simulink model "Electric_Machines_Design"  (R2021a)
settings: Solver=ode4  StartTime=0.0  StopTime=10.0  FixedStep=1e-6  RelTol=1e-3
libraries: spsSeriesRLCBranchLib x14, spsVoltageMeasurementLib x4, spsRMSLib x3, spsACVoltageSourceLib x1, spsAsynchronousMachineSIUnitsLib x1, spsPWMGenerator2LevelLib x1, spsTwoLevelConverterLib x1, spsUniversalBridgeLib x1, spsVariableRatioTransformerLib x1, spspowerguiLib x1
settings Model: Creator=SULEYMAN  LastModifiedBy=erena
settings DebuggingCC: UnconnectedInputMsg=none  UnconnectedOutputMsg=none  UnconnectedLineMsg=none
settings ModelReferenceCC: EnableRefExpFcnMdlSchedulingChecks=off
settings RTWCC: Description=Generic Real-Time Target  GPUComputeCapability=5.0  DLArmComputeVersion=20.02.1

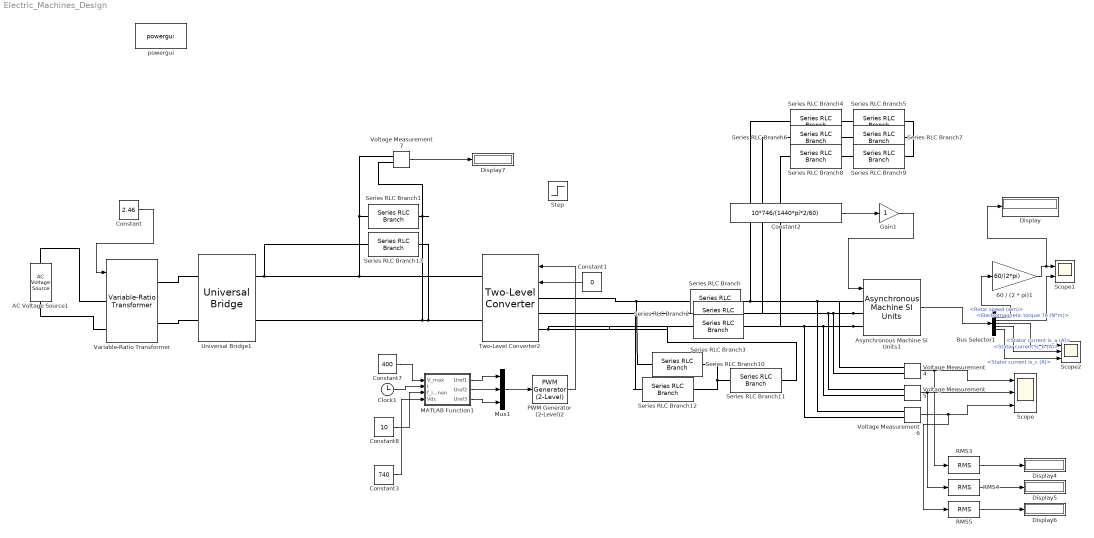
== system Electric_Machines_Design ==
  60 / (2 * pi)1 : Gain  Gain=60/(2*pi)
  AC Voltage Source1 : spsACVoltageSourceLib/AC Voltage Source  Amplitude=312  Phase=0  Frequency=50  SampleTime=0  Measurements=None  BusType=swing  Pref=10e3  Qref=0  Qmin=-inf  Qmax=+inf
  Asynchronous Machine SI Units1 : spsAsynchronousMachineSIUnitsLib/Asynchronous Machine SI Units  RotorType=Squirrel-cage  PresetModel="16:  10 HP (7.5KW)  400 V 50Hz 1440 RPM"  MechanicalLoad=Torque Tm  ShowDetailedParameters=on  ReferenceFrame=Rotor  Units=SI  MeasurementBus=off  NominalParameters=[7500 400 50]  VoltageRatio=1  Stator=[0.7384 0.003045]  Rotor=[0.7402 0.003045]  Cage1=[0.4155 0.002066]  Cage2=[0.4168 0.0003495]  Lm=0.1241  Mechanical=[0.0343 0.000503 2]  PolePairs=2  InitialConditions=[1 0 0 0 0 0 0 0]  SimulateSaturation=off  Saturation=[14.03593122, 27.81365428, 53.79336849, 72.68890987, 97.98006896, 148.6815601, 215.7428561, 302.9841135, 428.7778367 ; 230, 322, 414, 460, 506, 552, 598, 644, 690]  LoadFlowParameters=1492000  TsPowergui=0  TsBlock=-1  IterativeModel=Trapezoidal non iterative  IterativeDiscreteModel=Trapezoidal non iterative  Pmec=1.492e+006
  Bus Selector1 : BusSelector  OutputSignals=Mechanical.Rotor speed (wm),Mechanical.Electromagnetic torque Te (N*m),Stator measurements.Stator current is_a (A),Stator measurements.Stator current is_b (A),Stator measurements.Stator current is_c (A)
  Clock1 : Clock
  Constant : Constant  Value=2.46
  Constant1 : Constant  Value=0
  Constant2 : Constant  Value=10*746/(1440*pi*2/60)
  Constant3 : Constant  Value=740
  Constant7 : Constant  Value=400
  Constant8 : Constant  Value=10
  Display{,4..7} (5 alike) : Display
      Display6 settings: Decimation=50
  Gain1 : Gain
  MATLAB Function1 : MATLAB Function  TreatAsAtomicUnit=on
  Mux1 : Mux  Inputs=3
  PWM Generator (2-Level)2 : spsPWMGenerator2LevelLib/PWM Generator (2-Level)  ModulatorType=Three-phase bridge (6 pulses)  ModulatorMode=Unsynchronized  Fc=200*60  Pc=90  nF=27  MinMax="[ -1  1 ]"  SamplingTechnique=Natural  ModulatingSignals=off  m=0.8  Freq=60  Phase=0  Ts=1e-6  ShowCarrierOutport=off
  RMS3 : spsRMSLib/RMS  TrueRMS=off  Freq=10  RMSInit=0  Ts=0
  RMS4 : spsRMSLib/RMS  TrueRMS=off  Freq=10  RMSInit=0  Ts=0
  RMS5 : spsRMSLib/RMS  TrueRMS=off  Freq=10  RMSInit=0  Ts=0
  Scope : Scope  NumInputPorts=3
  Scope1 : Scope  NumInputPorts=2
  Scope2 : Scope  NumInputPorts=3
  Series RLC Branch : spsSeriesRLCBranchLib/Series RLC Branch  LConnTagsString=__new0  RConnTagsString=__new0  BranchType=L  Resistance=1  Inductance=3.5e-3  SetiL0=off  InitialCurrent=0  Capacitance=1e-6  Setx0=off  InitialVoltage=0  Measurements=None
  Series RLC Branch1 : spsSeriesRLCBranchLib/Series RLC Branch  LConnTagsString=__new0  RConnTagsString=__new0  BranchType=C  Resistance=1  Inductance=1e-3  SetiL0=off  InitialCurrent=0  Capacitance=4700e-6  Setx0=off  InitialVoltage=0  Measurements=None
  Series RLC Branch10 : spsSeriesRLCBranchLib/Series RLC Branch  LConnTagsString=__new0  RConnTagsString=__new0  BranchType=R  Resistance=1e5  Inductance=1e-3  SetiL0=off  InitialCurrent=0  Capacitance=1e-6  Setx0=off  InitialVoltage=0  Measurements=None
  Series RLC Branch11 : spsSeriesRLCBranchLib/Series RLC Branch  LConnTagsString=__new0  RConnTagsString=__new0  BranchType=R  Resistance=1e5  Inductance=1e-3  SetiL0=off  InitialCurrent=0  Capacitance=1e-6  Setx0=off  InitialVoltage=0  Measurements=None
  Series RLC Branch12 : spsSeriesRLCBranchLib/Series RLC Branch  LConnTagsString=__new0  RConnTagsString=__new0  BranchType=R  Resistance=1e5  Inductance=1e-3  SetiL0=off  InitialCurrent=0  Capacitance=1e-6  Setx0=off  InitialVoltage=0  Measurements=None
  Series RLC Branch13 : spsSeriesRLCBranchLib/Series RLC Branch  LConnTagsString=__new0  RConnTagsString=__new0  BranchType=C  Resistance=1  Inductance=1e-3  SetiL0=off  InitialCurrent=0  Capacitance=4700e-6  Setx0=off  InitialVoltage=0  Measurements=None
  Series RLC Branch2 : spsSeriesRLCBranchLib/Series RLC Branch  LConnTagsString=__new0  RConnTagsString=__new0  BranchType=L  Resistance=1  Inductance=3.5e-3  SetiL0=off  InitialCurrent=0  Capacitance=1e-6  Setx0=off  InitialVoltage=0  Measurements=None
  Series RLC Branch3 : spsSeriesRLCBranchLib/Series RLC Branch  LConnTagsString=__new0  RConnTagsString=__new0  BranchType=L  Resistance=1  Inductance=3.5e-3  SetiL0=off  InitialCurrent=0  Capacitance=1e-6  Setx0=off  InitialVoltage=0  Measurements=None
  Series RLC Branch4 : spsSeriesRLCBranchLib/Series RLC Branch  LConnTagsString=__new0  RConnTagsString=__new0  BranchType=C  Resistance=1  Inductance=1e-3  SetiL0=off  InitialCurrent=0  Capacitance=6.6e-6  Setx0=off  InitialVoltage=0  Measurements=None
  Series RLC Branch5 : spsSeriesRLCBranchLib/Series RLC Branch  LConnTagsString=__new0  RConnTagsString=__new0  BranchType=R  Resistance=5  Inductance=1e-3  SetiL0=off  InitialCurrent=0  Capacitance=1e-6  Setx0=off  InitialVoltage=0  Measurements=None
  Series RLC Branch6 : spsSeriesRLCBranchLib/Series RLC Branch  LConnTagsString=__new0  RConnTagsString=__new0  BranchType=C  Resistance=1  Inductance=1e-3  SetiL0=off  InitialCurrent=0  Capacitance=6.6e-6  Setx0=off  InitialVoltage=0  Measurements=None
  Series RLC Branch7 : spsSeriesRLCBranchLib/Series RLC Branch  LConnTagsString=__new0  RConnTagsString=__new0  BranchType=R  Resistance=5  Inductance=1e-3  SetiL0=off  InitialCurrent=0  Capacitance=1e-6  Setx0=off  InitialVoltage=0  Measurements=None
  Series RLC Branch8 : spsSeriesRLCBranchLib/Series RLC Branch  LConnTagsString=__new0  RConnTagsString=__new0  BranchType=C  Resistance=1  Inductance=1e-3  SetiL0=off  InitialCurrent=0  Capacitance=6.6e-6  Setx0=off  InitialVoltage=0  Measurements=None
  Series RLC Branch9 : spsSeriesRLCBranchLib/Series RLC Branch  LConnTagsString=__new0  RConnTagsString=__new0  BranchType=R  Resistance=5  Inductance=1e-3  SetiL0=off  InitialCurrent=0  Capacitance=1e-6  Setx0=off  InitialVoltage=0  Measurements=None
  Step : Step  Time=2.5  After=10*746/(1440*pi*2/60)  SampleTime=0
  Two-Level Converter2 : spsTwoLevelConverterLib/Two-Level Converter  ModelType=Switching devices  Ron=1e-3  Rs=1e6  Cs=inf  Vforward=[0,0]  Ron_Diode=1e-3  Rs_Diode=1e6  Cs_Diode=inf  Vf_Diode=1e-3  Rs_CurrentSource=inf
      settings: SourceProductBaseCode=PS
  Universal Bridge1 : spsUniversalBridgeLib/Universal Bridge  Arms=2  SnubberResistance=1e5  SnubberCapacitance=inf  Device=Diodes  Ron=1e-3  Lon=0  ForwardVoltages="[  0  0  ]"  ForwardVoltage=0  GTOparameters=[ 10e-6 , 20e-6 ]  IGBTparameters=[ 1e-6 , 2e-6 ]  Measurements=None  Measurements_2=None  converterType=Rectifier
  Variable-Ratio Transformer : spsVariableRatioTransformerLib/Variable-Ratio Transformer
      settings: SourceProductBaseCode=PS
  Voltage Measurement{4..7} (4 alike) : spsVoltageMeasurementLib/Voltage Measurement  PhasorSimulation=off  OutputType=Complex  PSBequivalent=0
  powergui : spspowerguiLib/powergui  Priority=1  SimulationMode=Discrete  SampleTime=1e-6  frequency=50  Iterations=50  frequencyindice=50  Pbase=100e6  ErrMax=1e-4  UnitsV=kV  UnitsW=MW  buscounter=0  FunctionMessages=off  echomessages=off  EnableUseOfTLC=off  CurrentSourceSwitches=off  DisableSnubberDevices=off  DisableRonSwitches=off  DisableVfSwitches=off  DisplayEquations=off  AutomaticDiscreteSolvers=off  SolverType=Tustin/Backward Euler (TBE)  Interpol=off  ExternalGateDelay=off  methode=off  Ts=100  x0status=blocks  SPID=on  SwTol=0  HookPort=off  NonlinearTolerance=1e-4  nMaxIteration=100  ContinueOnMaxIteration=off  RestoreLinks=warning  ResistiveCurrentMeasurement=off  Frange=[0:2:500]  Ylog=off  Xlog=on  ShowGrid=off  save=off  variable=ZData  structure=0  ZoomFFT=off  StartTime=0.0  cycles=1  DisplayStyle=1  fundamental=60  FreqAxis=off  MaxFrequency=1000  frequencyindicesteady=1  RmsSteady=1  display=off
  wires:
  Asynchronous Machine SI Units1/1 -> Bus Selector1/1
  MATLAB Function1/1(Uref1) -> Mux1/1
  Voltage Measurement7/1 -> Display7/1
  Bus Selector1/4 -> Scope2/2  "<Stator current is_b (A)>"
  60 / (2 * pi)1/1 -> Display/1, Scope1/1
  Bus Selector1/3 -> Scope2/1  "<Stator current is_a (A)>"
  Bus Selector1/2 -> Scope1/2  "<Electromagnetic torque Te (N*m)>"
  Constant1/1 -> Two-Level Converter2/2
  PWM Generator (2-Level)2/1 -> Two-Level Converter2/1
  MATLAB Function1/3(Uref3) -> Mux1/3
  Bus Selector1/5 -> Scope2/3  "<Stator current is_c (A)>"
  Clock1/1 -> MATLAB Function1/2(t)
  Bus Selector1/1 -> 60 / (2 * pi)1/1  "<Rotor speed (wm)>"
  Constant7/1 -> MATLAB Function1/1(V_max)
  Mux1/1 -> PWM Generator (2-Level)2/1
  Gain1/1 -> Asynchronous Machine SI Units1/1
  MATLAB Function1/2(Uref2) -> Mux1/2
  Constant/1 -> Variable-Ratio Transformer/1
  RMS3/1 -> Display4/1
  RMS4/1 -> Display5/1
  RMS5/1 -> Display6/1
  Voltage Measurement4/1 -> Scope/1, RMS3/1
  Voltage Measurement5/1 -> Scope/2, RMS4/1
  Voltage Measurement6/1 -> RMS5/1, Scope/3
  Constant8/1 -> MATLAB Function1/3(f_istenen)
  Constant3/1 -> MATLAB Function1/4(Vdc)
  Constant2/1 -> Gain1/1
  connections:
  Asynchronous Machine SI Units1/LConn3 -- Voltage Measurement6/LConn2 -- Series RLC Branch8/LConn1 -- Series RLC Branch3/RConn1 -- Voltage Measurement5/LConn2
  Asynchronous Machine SI Units1/LConn1 -- Voltage Measurement4/LConn1 -- Voltage Measurement6/LConn1 -- Series RLC Branch4/LConn1 -- Series RLC Branch/RConn1
  Series RLC Branch1/RConn1 -- Voltage Measurement7/LConn2 -- Series RLC Branch13/RConn1 -- Two-Level Converter2/RConn2 -- Universal Bridge1/RConn2
  Asynchronous Machine SI Units1/LConn2 -- Voltage Measurement4/LConn2 -- Series RLC Branch6/LConn1 -- Series RLC Branch2/RConn1 -- Voltage Measurement5/LConn1
  AC Voltage Source1/RConn1 -- Variable-Ratio Transformer/LConn1
  AC Voltage Source1/LConn1 -- Variable-Ratio Transformer/LConn2
  Universal Bridge1/LConn1 -- Variable-Ratio Transformer/RConn1
  Variable-Ratio Transformer/RConn2 -- Universal Bridge1/LConn2
  Series RLC Branch/LConn1 -- Series RLC Branch10/LConn1 -- Two-Level Converter2/LConn1
  Two-Level Converter2/LConn2 -- Series RLC Branch12/LConn1 -- Series RLC Branch2/LConn1
  Two-Level Converter2/LConn3 -- Series RLC Branch11/LConn1 -- Series RLC Branch3/LConn1
  Series RLC Branch4/RConn1 -- Series RLC Branch5/LConn1
  Series RLC Branch6/RConn1 -- Series RLC Branch7/LConn1
  Series RLC Branch8/RConn1 -- Series RLC Branch9/LConn1
  Series RLC Branch5/RConn1 -- Series RLC Branch9/RConn1 -- Series RLC Branch7/RConn1
  Series RLC Branch10/RConn1 -- Series RLC Branch11/RConn1 -- Series RLC Branch12/RConn1
  Series RLC Branch1/LConn1 -- Voltage Measurement7/LConn1 -- Series RLC Branch13/LConn1 -- Universal Bridge1/RConn1 -- Two-Level Converter2/RConn1

== matlab function Electric_Machines_Design/MATLAB Function1 ==
  settings: updateMethod=DISCRETE
  data: V_max input; t input; f_istenen input; Uref1 output; Uref2 output; Uref3 output; Vdc input
function [Uref1, Uref2, Uref3] = fcn(V_max, t, f_istenen, Vdc)

    % Hertz başına 8 Volt artış kuralı
    volt_per_hz = 8;
    V_ref = volt_per_hz * f_istenen; 

    % Üst sınır kontrolü
    if V_ref > V_max, V_ref = V_max; end
    if V_ref < 0, V_ref = 0; end

    % --- DINAMIK VOLTAJ REGLASYONU ---
    % Kapasitörün anlık dalgalanan voltajını (535-548V) işleme alıyoruz.
    % Simülasyonun ilk başında sıfır gelme riskine karşı güvenlik sınırı:
    if Vdc < 10
        Vdc_anlik = 540;
    else
        Vdc_anlik = Vdc; % Kapasitörden gelen anlık dalgalı voltaj
    end

    % Hat-Hat RMS -> Faz-Nötr Tepe Değeri Dönüşümü
    V_faz_tepe = (V_ref * sqrt(2)) / sqrt(3);
    
    % Modülasyon indeksi artık sabit bir sayıya değil, anlık Vdc'ye bölünüyor!
    K_yeni = (2 * V_faz_tepe) / Vdc_anlik;
    % ----------------------------------

    % Açı Hesabı
    theta = mod(2 * pi * f_istenen * t, 2 * pi); 

    % Temel sinüs dalgaları
    u1 = K_yeni * sin(theta);
    u2 = K_yeni * sin(theta - 2*pi/3);
    u3 = K_yeni * sin(theta + 2*pi/3);

    % Space Vector (SVPWM) Etkisi için 3. Harmonik Enjeksiyonu
    % Bu kısım voltajın 346V bariyerini aşmasını sağlar.
    v_ofset = 0.5 * (max([u1, u2, u3]) + min([u1, u2, u3]));
    
    Uref1 = u1 - v_ofset;
    Uref2 = u2 - v_ofset;
    Uref3 = u3 - v_ofset;

    % Satürasyon Sınırları
    if Uref1 > 1, Uref1 = 1; elseif Uref1 < -1, Uref1 = -1; end
    if Uref2 > 1, Uref2 = 1; elseif Uref2 < -1, Uref2 = -1; end
    if Uref3 > 1, Uref3 = 1; elseif Uref3 < -1, Uref3 = -1; end

end
